simulink model "DroneModelv7_FTX"  (R2025a)
settings: Solver=ode4  StartTime=10  StopTime=60  FixedStep=0.001  RelTol=1e-3
undefined symbols (not defined in the file): ACT_MAP, alpha_vec, alpha_vec_control, beta_vec, bref, Cl0, Clda, Cldr, Cm0, Cmda, Cmde, Cmdr, Cn0, Cnda, Cndr, CX0, CXda, CXde, CXdr, CY0, CYda, CYdr, CZ0, CZda, CZde, CZdr, DEMAND0, DEMAND1, DMP_P, EST_BLEND, EST_P, EST_TS, Kalpha, Kbeta, Kp, Kphi, Kq, Kr, mass, RT_LIM_ALPHA, RT_LIM_BETA, RT_LIM_PHI, RT_PA_SCALE, RT_PB_SCALE, RT_PP_SCALE, RT_SURF_LIM, SENS_P, T_STEP, Tc, x_cg, y_cg, z_cg
libraries: aerolibconvert2 x6, aerolibasang x3, slpidlib x3, aerolibobsolete x1, aerolibadyn x1, aerolibatmos2 x1
Description:
  | DroneModelv7_RT - re-tunable controller, generated by
  | tools/build_rt_v7.m from DroneModelv7_EST.
  | 
  | Adds output limits, clamping anti-windup and surface saturation, and
  | exposes the fixed P gains as scale factors so the loop can be re-tuned
  | against a plant that includes the sensor and estimator models.
  | 
  | Outports 1-13 keep the indices they have in DroneModelv7_EST; 14 and 15
  | are the post-saturation surface deflections. 7 and 8 remain the
  | pre-saturation COMMAND, which is the diagnostic worth keeping.
settings Model: SimulationMode=accelerator  Creator=Avery  LastModifiedBy=avery
settings DataIOCC: ExternalInput=getinputstruct(op1)  InitialState=getstatestruct(op1)
settings OptimizationCC: BlockReduction=off  ConditionallyExecuteInputs=off
settings DebuggingCC: UnconnectedInputMsg=error  UnconnectedOutputMsg=warning  UnconnectedLineMsg=warning
settings RTWCC: GPUComputeCapability=3.5

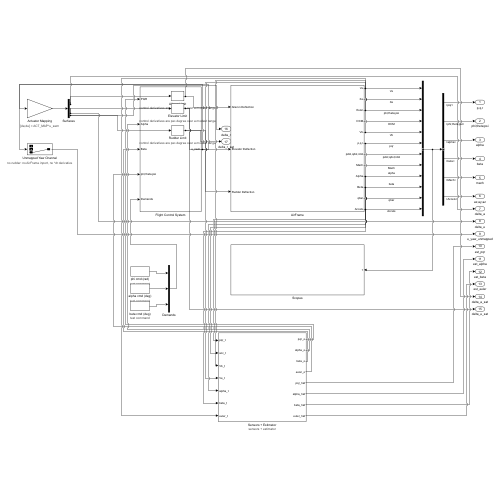
[thumbnail: Simulink's stored preview of the top-level diagram]
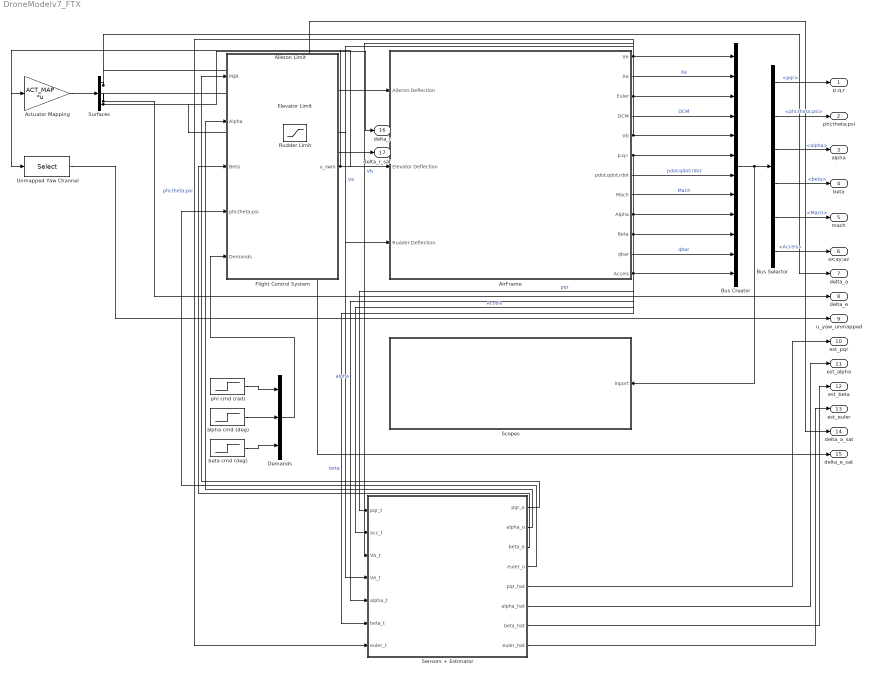
== system DroneModelv7_FTX ==
  Actuator Mapping : Gain  Gain=ACT_MAP  Multiplication=Matrix(K*u)
      settings: AttributesFormatString=[da;de] = ACT_MAP*u_swm
  Aileron Limit : Saturate  UpperLimit=RT_SURF_LIM  LowerLimit=-RT_SURF_LIM
      settings: AttributesFormatString=control derivatives are per-degree over a modest range
  AirFrame : Subsystem
  Bus Creator : BusCreator  Inputs=12
  Bus Selector : BusSelector  OutputSignals=pqr,phi;theta;psi,alpha,beta,Mach,Accels
  Demands : Mux  Inputs=3
  Elevator Limit : Saturate  UpperLimit=RT_SURF_LIM  LowerLimit=-RT_SURF_LIM
      settings: AttributesFormatString=control derivatives are per-degree over a modest range
  Flight Control System : Subsystem
  Rudder Limit : Saturate  UpperLimit=RT_SURF_LIM  LowerLimit=-RT_SURF_LIM
      settings: AttributesFormatString=control derivatives are per-degree over a modest range
  Scopes : Subsystem
  Sensors + Estimator : Subsystem
      settings: AttributesFormatString=sensors + estimator
  Surfaces : Demux  Outputs=3
  Unmapped Yaw Channel : Selector  InputPortWidth=3  IndexOptions=Index vector (dialog)  Indices=[3]  OutputSizes=1
      settings: AttributesFormatString=no rudder: no AirFrame inport, no *dr derivative
  alpha cmd (deg) : Step  Time=T_STEP(2)  Before=DEMAND0(2)  After=DEMAND1(2)  SampleTime=0
      settings: AttributesFormatString=test command
  beta cmd (deg) : Step  Time=T_STEP(3)  Before=DEMAND0(3)  After=DEMAND1(3)  SampleTime=0
      settings: AttributesFormatString=test command
  phi cmd (rad) : Step  Time=T_STEP(1)  Before=DEMAND0(1)  After=DEMAND1(1)  SampleTime=0
      settings: AttributesFormatString=test command
  p,q,r : Outport
  phi;theta;psi : Outport  Port=2
  alpha : Outport  Port=3
  beta : Outport  Port=4
  mach : Outport  Port=5
  ax;ay;az : Outport  Port=6
  delta_a : Outport  Port=7
  delta_e : Outport  Port=8
  u_yaw_unmapped : Outport  Port=9
  est_pqr : Outport  Port=10
  est_alpha : Outport  Port=11
  est_beta : Outport  Port=12
  est_euler : Outport  Port=13
  delta_a_sat : Outport  Port=14
  delta_e_sat : Outport  Port=15
  delta_r : Outport  Port=16
  delta_r_sat : Outport  Port=17
  wires:
  AirFrame/12(Accels) -> Bus Creator/12, Sensors + Estimator/2(acc_t)  "Accels"
  AirFrame/11(qbar) -> Bus Creator/11  "qbar"
  AirFrame/10(Beta) -> Bus Creator/10, Sensors + Estimator/6(beta_t)  "beta"
  AirFrame/9(Alpha) -> Bus Creator/9, Sensors + Estimator/5(alpha_t)  "alpha"
  AirFrame/8(Mach) -> Bus Creator/8  "Mach"
  AirFrame/7(pdot,qdot,rdot) -> Bus Creator/7  "pdot;qdot;rdot"
  AirFrame/6(p,q,r) -> Bus Creator/6, Sensors + Estimator/1(pqr_t)  "pqr"
  AirFrame/5(Vb) -> Bus Creator/5, Sensors + Estimator/3(Vb_t)  "Vb"
  AirFrame/4(DCM) -> Bus Creator/4  "DCM"
  AirFrame/3(Euler) -> Bus Creator/3, Sensors + Estimator/7(euler_t)  "phi;theta;psi"
  AirFrame/2(Xe) -> Bus Creator/2  "Xe"
  AirFrame/1(Ve) -> Bus Creator/1, Sensors + Estimator/4(Ve_t)  "Ve"
  Bus Selector/1 -> p,q,r/1  "<pqr>"
  Bus Selector/2 -> phi;theta;psi/1  "<phi;theta;psi>"
  Bus Selector/3 -> alpha/1  "<alpha>"
  Bus Selector/5 -> mach/1  "<Mach>"
  Bus Selector/6 -> ax;ay;az/1  "<Accels>"
  Bus Selector/4 -> beta/1  "<beta>"
  Bus Creator/1 -> Scopes/1(Inport), Bus Selector/1
  phi cmd (rad)/1 -> Demands/1
  alpha cmd (deg)/1 -> Demands/2
  beta cmd (deg)/1 -> Demands/3
  Demands/1 -> Flight Control System/5(Demands)
  Flight Control System/1(u_swm) -> Actuator Mapping/1, Unmapped Yaw Channel/1
  Actuator Mapping/1 -> Surfaces/1
  Surfaces/1 -> delta_a/1, Aileron Limit/1
  Surfaces/2 -> delta_e/1, Elevator Limit/1
  Unmapped Yaw Channel/1 -> u_yaw_unmapped/1
  Sensors + Estimator/1(pqr_o) -> Flight Control System/1("PQR ")
  Sensors + Estimator/2(alpha_o) -> Flight Control System/2(Alpha)
  Sensors + Estimator/3(beta_o) -> Flight Control System/3(Beta)
  Sensors + Estimator/4(euler_o) -> Flight Control System/4(phi;theta;psi)
  Sensors + Estimator/5(pqr_hat) -> est_pqr/1
  Sensors + Estimator/6(alpha_hat) -> est_alpha/1
  Sensors + Estimator/7(beta_hat) -> est_beta/1
  Sensors + Estimator/8(euler_hat) -> est_euler/1
  Aileron Limit/1 -> AirFrame/1(Aileron Deflection), delta_a_sat/1
  Elevator Limit/1 -> AirFrame/2(Elevator Deflection), delta_e_sat/1
  Surfaces/3 -> Rudder Limit/1, delta_r/1
  Rudder Limit/1 -> AirFrame/3(Rudder Deflection), delta_r_sat/1

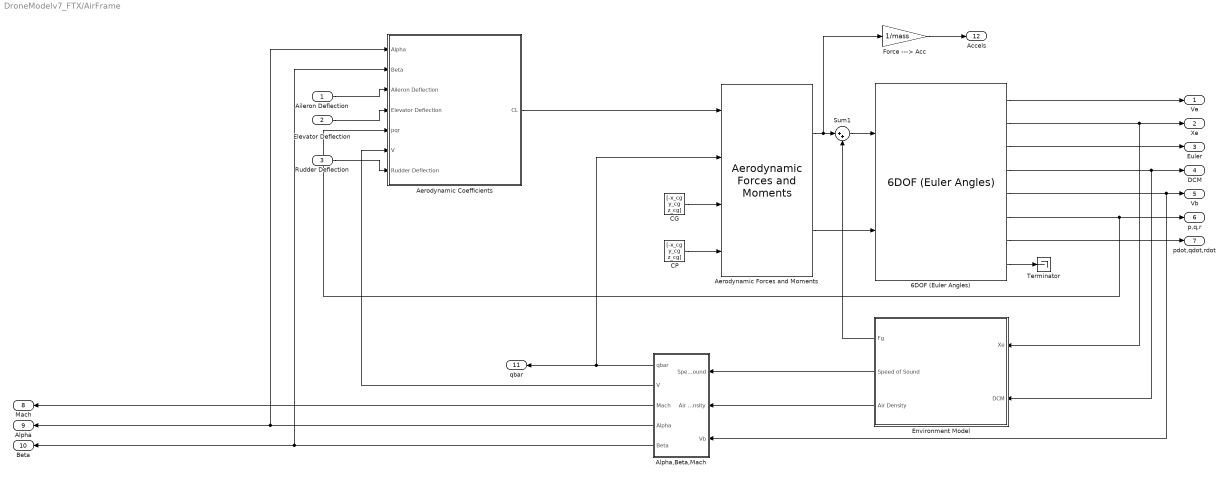
== system DroneModelv7_FTX/AirFrame ==
  Aileron Deflection : Inport  Unit=deg
  Elevator Deflection : Inport  Port=2  Unit=deg
  Rudder Deflection : Inport  Port=3
  6DOF (Euler Angles) : aerolibobsolete/6DOF (Euler Angles)  units=Metric (MKS)  mtype=Fixed  rep=Euler Angles  xme_0=init_pos_inertial  Vm_0=init_velo_body  eul_0=init_euler_orien  pm_0=init_body_rot  mass_0=mass  mass_e=0.5  mass_f=2.0  inertia=Inertia  inertia_e=eye(3)  inertia_f=2*eye(3)  k_quat=1.0  vre_flag=on  abi_flag=off  aMode=0  xme_statename=''  Vm_statename=''  eul_statename=''  quat_statename=''  pm_statename=''  mass_statename=''
  "Aerodynamic Forces and Moments " : aerolibadyn/Aerodynamic Forces and Moments   inputAxes=Body  outputForceAxes=Body  outputMomentAxes=Body  S=Sref  b=bref  cbar=cref
  Aerodynamic Coefficients : Subsystem
  Alpha,Beta,Mach : Subsystem
  CG : Constant  Value=[-x_cg y_cg z_cg]
  CP : Constant  Value=[-x_cg y_cg z_cg]
  Environment Model : Subsystem
  Force ---> Acc : Gain  Gain=1/mass  SaturateOnIntegerOverflow=on  OutDataTypeStr=Inherit: Same as input  ParamDataTypeStr=Inherit: Same as input
  Sum1 : Sum  Inputs=|++  SaturateOnIntegerOverflow=on
  Terminator : Terminator
  Ve : Outport  Unit=m/s
  Xe : Outport  Port=2  Unit=meter
  Euler : Outport  Port=3  Unit=rad
  DCM : Outport  Port=4
  Vb : Outport  Port=5  Unit=m/second
  p,q,r : Outport  Port=6  Unit=rad/second
  pdot,qdot,rdot : Outport  Port=7
  Mach : Outport  Port=8
  Alpha : Outport  Port=9  Unit=rad
  Beta : Outport  Port=10  Unit=rad
  qbar : Outport  Port=11  Unit=Pa
  Accels : Outport  Port=12  Unit=m/s^2
  wires:
  6DOF (Euler Angles)/6 -> Aerodynamic Coefficients/5(pqr), p,q,r/1
  6DOF (Euler Angles)/4 -> DCM/1, Environment Model/2(DCM)
  6DOF (Euler Angles)/2 -> Xe/1, Environment Model/1(Xe)
  6DOF (Euler Angles)/5 -> Alpha,Beta,Mach/3(Vb), Vb/1
  "Aerodynamic Forces and Moments "/1 -> Force ---> Acc/1, Sum1/1
  6DOF (Euler Angles)/3 -> Euler/1
  6DOF (Euler Angles)/1 -> Ve/1
  CP/1 -> "Aerodynamic Forces and Moments "/4
  Alpha,Beta,Mach/1(qbar) -> qbar/1, "Aerodynamic Forces and Moments "/2
  CG/1 -> "Aerodynamic Forces and Moments "/3
  Alpha,Beta,Mach/4(Alpha) -> Aerodynamic Coefficients/1(Alpha), Alpha/1
  6DOF (Euler Angles)/8 -> Terminator/1
  "Aerodynamic Forces and Moments "/2 -> 6DOF (Euler Angles)/2
  6DOF (Euler Angles)/7 -> pdot,qdot,rdot/1
  Alpha,Beta,Mach/2(V) -> Aerodynamic Coefficients/6(V)
  Environment Model/1(Fg) -> Sum1/2
  Sum1/1 -> 6DOF (Euler Angles)/1
  Force ---> Acc/1 -> Accels/1
  Alpha,Beta,Mach/5(Beta) -> Aerodynamic Coefficients/2(Beta), Beta/1
  Alpha,Beta,Mach/3(Mach) -> Mach/1
  Environment Model/2(Speed of Sound) -> Alpha,Beta,Mach/1(Speed of Sound)
  Environment Model/3(Air Density) -> Alpha,Beta,Mach/2(Air Density)
  Aerodynamic Coefficients/1(CL) -> "Aerodynamic Forces and Moments "/1
  Elevator Deflection/1 -> Aerodynamic Coefficients/4(Elevator Deflection)
  Aileron Deflection/1 -> Aerodynamic Coefficients/3(Aileron Deflection)
  Rudder Deflection/1 -> Aerodynamic Coefficients/7(Rudder Deflection)

== system DroneModelv7_FTX/Flight Control System ==
  "PQR " : Inport
  Alpha : Inport  Port=2
  Beta : Inport  Port=3
  phi;theta;psi : Inport  Port=4
  Demands : Inport  Port=5
      settings: AttributesFormatString=test command vector
  Angle Conversion : aerolibconvert2/Angle Conversion  IU=rad  OU=deg
  Angle Conversion1 : aerolibconvert2/Angle Conversion  IU=rad  OU=deg
  Controller : Subsystem
  Selector : Selector  InputPortWidth=3  IndexOptions=Index vector (dialog)  Indices=[1]  OutputSizes=1
  u_swm : Outport
  wires:
  "PQR "/1 -> Controller/5(Rates)
  Alpha/1 -> Angle Conversion/1
  Beta/1 -> Angle Conversion1/1
  Angle Conversion1/1 -> Controller/3(Beta)
  Angle Conversion/1 -> Controller/2(Alpha)
  phi;theta;psi/1 -> Selector/1
  Selector/1 -> Controller/1(Phi)  "phi"
  Demands/1 -> Controller/4(Demands)
  Controller/1(u_swm) -> u_swm/1

== system DroneModelv7_FTX/Scopes ==
  Inport : Inport
  Angle Conversion : aerolibconvert2/Angle Conversion  IU=rad  OU=deg
  Angle Conversion1 : aerolibconvert2/Angle Conversion  IU=rad  OU=deg
  Bus Selector : BusSelector  OutputSignals=alpha,beta,Mach,pqr,phi;theta;psi,Xe,Vb
  Scope : Scope  NumInputPorts=3
      settings: ActiveDisplayYMinimum=2.14483  ActiveDisplayYMaximum=2.82837
  Scope1 : Scope  NumInputPorts=4
      settings: ActiveDisplayYMinimum=-0.1468  ActiveDisplayYMaximum=0.04977
  wires:
  Bus Selector/1 -> Angle Conversion/1  "<alpha>"
  Bus Selector/2 -> Angle Conversion1/1  "<beta>"
  Bus Selector/3 -> Scope/3  "<Mach>"
  Bus Selector/4 -> Scope1/1  "<pqr>"
  Bus Selector/5 -> Scope1/2  "<phi;theta;psi>"
  Bus Selector/6 -> Scope1/3  "<Xe>"
  Inport/1 -> Bus Selector/1
  Angle Conversion1/1 -> Scope/2  "beta"
  Angle Conversion/1 -> Scope/1  "alpha"
  Bus Selector/7 -> Scope1/4  "<Vb>"

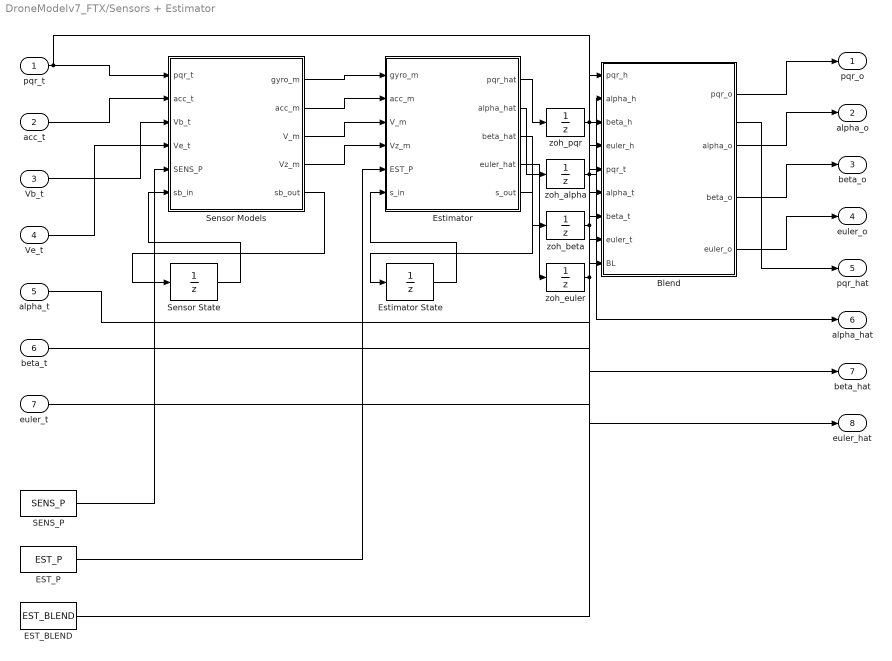
== system DroneModelv7_FTX/Sensors + Estimator ==
  pqr_t : Inport
  acc_t : Inport  Port=2
  Vb_t : Inport  Port=3
  Ve_t : Inport  Port=4
  alpha_t : Inport  Port=5
  beta_t : Inport  Port=6
  euler_t : Inport  Port=7
  Blend : MATLAB Function  TreatAsAtomicUnit=on
  EST_BLEND : Constant  Value=EST_BLEND
  EST_P : Constant  Value=EST_P
  Estimator : MATLAB Function  TreatAsAtomicUnit=on
  Estimator State : UnitDelay  InitialCondition=zeros(10,1)  SampleTime=EST_TS  HasFrameUpgradeWarning=on
  SENS_P : Constant  Value=SENS_P
  Sensor Models : MATLAB Function  TreatAsAtomicUnit=on
  Sensor State : UnitDelay  InitialCondition=zeros(4,1)  SampleTime=EST_TS  HasFrameUpgradeWarning=on
  zoh_alpha : UnitDelay  SampleTime=EST_TS  HasFrameUpgradeWarning=on
      settings: AttributesFormatString=sensor + compute latency, 1 sample
  zoh_beta : UnitDelay  SampleTime=EST_TS  HasFrameUpgradeWarning=on
      settings: AttributesFormatString=sensor + compute latency, 1 sample
  zoh_euler : UnitDelay  SampleTime=EST_TS  HasFrameUpgradeWarning=on
      settings: AttributesFormatString=sensor + compute latency, 1 sample
  zoh_pqr : UnitDelay  SampleTime=EST_TS  HasFrameUpgradeWarning=on
      settings: AttributesFormatString=sensor + compute latency, 1 sample
  pqr_o : Outport
  alpha_o : Outport  Port=2
  beta_o : Outport  Port=3
  euler_o : Outport  Port=4
  pqr_hat : Outport  Port=5
  alpha_hat : Outport  Port=6
  beta_hat : Outport  Port=7
  euler_hat : Outport  Port=8
  wires:
  pqr_t/1 -> Sensor Models/1(pqr_t), Blend/5(pqr_t)
  acc_t/1 -> Sensor Models/2(acc_t)
  Vb_t/1 -> Sensor Models/3(Vb_t)
  Ve_t/1 -> Sensor Models/4(Ve_t)
  SENS_P/1 -> Sensor Models/5(SENS_P)
  Sensor State/1 -> Sensor Models/6(sb_in)
  Sensor Models/5(sb_out) -> Sensor State/1
  Sensor Models/1(gyro_m) -> Estimator/1(gyro_m)
  Sensor Models/2(acc_m) -> Estimator/2(acc_m)
  Sensor Models/3(V_m) -> Estimator/3(V_m)
  Sensor Models/4(Vz_m) -> Estimator/4(Vz_m)
  EST_P/1 -> Estimator/5(EST_P)
  Estimator State/1 -> Estimator/6(s_in)
  Estimator/5(s_out) -> Estimator State/1
  Estimator/1(pqr_hat) -> zoh_pqr/1
  Estimator/2(alpha_hat) -> zoh_alpha/1
  Estimator/3(beta_hat) -> zoh_beta/1
  Estimator/4(euler_hat) -> zoh_euler/1
  zoh_pqr/1 -> Blend/1(pqr_h), pqr_hat/1
  zoh_alpha/1 -> Blend/2(alpha_h), alpha_hat/1
  zoh_beta/1 -> Blend/3(beta_h), beta_hat/1
  zoh_euler/1 -> Blend/4(euler_h), euler_hat/1
  alpha_t/1 -> Blend/6(alpha_t)
  beta_t/1 -> Blend/7(beta_t)
  euler_t/1 -> Blend/8(euler_t)
  EST_BLEND/1 -> Blend/9(BL)
  Blend/1(pqr_o) -> pqr_o/1
  Blend/2(alpha_o) -> alpha_o/1
  Blend/3(beta_o) -> beta_o/1
  Blend/4(euler_o) -> euler_o/1

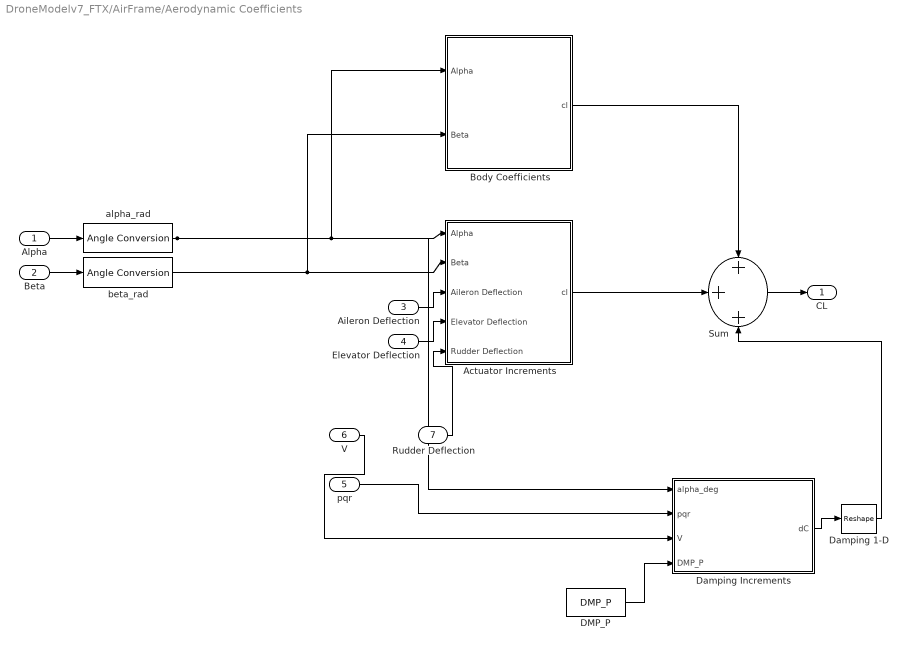
== system DroneModelv7_FTX/AirFrame/Aerodynamic Coefficients ==
  Alpha : Inport
  Beta : Inport  Port=2
  Aileron Deflection : Inport  Port=3
  Elevator Deflection : Inport  Port=4
  pqr : Inport  Port=5
  V : Inport  Port=6
  Rudder Deflection : Inport  Port=7
  Actuator Increments : Subsystem
  Body Coefficients : Subsystem
  DMP_P : Constant  Value=DMP_P
  Damping 1-D : Reshape
  Damping Increments : MATLAB Function  TreatAsAtomicUnit=on
  Sum : Sum  Inputs=+++  InputSameDT=on  SaturateOnIntegerOverflow=on  OutDataTypeStr=Inherit: Same as first input
  alpha_rad : aerolibconvert2/Angle Conversion  IU=rad  OU=deg
  beta_rad : aerolibconvert2/Angle Conversion  IU=rad  OU=deg
  CL : Outport
  wires:
  Elevator Deflection/1 -> Actuator Increments/4(Elevator Deflection)
  Beta/1 -> beta_rad/1
  Alpha/1 -> alpha_rad/1
  Body Coefficients/1(cl) -> Sum/1
  Aileron Deflection/1 -> Actuator Increments/3(Aileron Deflection)
  Actuator Increments/1(cl) -> Sum/2
  Sum/1 -> CL/1
  alpha_rad/1 -> Body Coefficients/1(Alpha), Actuator Increments/1(Alpha), Damping Increments/1(alpha_deg)
  beta_rad/1 -> Body Coefficients/2(Beta), Actuator Increments/2(Beta)
  pqr/1 -> Damping Increments/2(pqr)
  V/1 -> Damping Increments/3(V)
  DMP_P/1 -> Damping Increments/4(DMP_P)
  Damping Increments/1(dC) -> Damping 1-D/1
  Damping 1-D/1 -> Sum/3
  Rudder Deflection/1 -> Actuator Increments/5(Rudder Deflection)

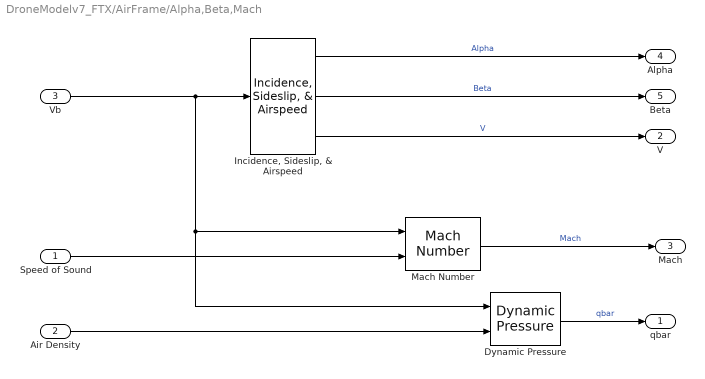
== system DroneModelv7_FTX/AirFrame/Alpha,Beta,Mach ==
  Speed of Sound : Inport
  Air Density : Inport  Port=2
  Vb : Inport  Port=3  PortDimensions=3
  Dynamic Pressure : aerolibasang/Dynamic Pressure
  "Incidence, Sideslip, & Airspeed" : aerolibasang/Incidence, Sideslip, & Airspeed
  Mach Number : aerolibasang/Mach Number
  qbar : Outport  Unit=Pa  InitialOutput=0  VectorParamsAs1DForOutWhenUnconnected=off
  V : Outport  Port=2  Unit=m/s  VectorParamsAs1DForOutWhenUnconnected=off
  Mach : Outport  Port=3  VectorParamsAs1DForOutWhenUnconnected=off
  Alpha : Outport  Port=4  Unit=rad  VectorParamsAs1DForOutWhenUnconnected=off
  Beta : Outport  Port=5  Unit=rad  VectorParamsAs1DForOutWhenUnconnected=off
  wires:
  Air Density/1 -> Dynamic Pressure/2
  "Incidence, Sideslip, & Airspeed"/2 -> Beta/1  "Beta"
  "Incidence, Sideslip, & Airspeed"/1 -> Alpha/1  "Alpha"
  Vb/1 -> Dynamic Pressure/1, Mach Number/1, "Incidence, Sideslip, & Airspeed"/1
  Mach Number/1 -> Mach/1  "Mach"
  Dynamic Pressure/1 -> qbar/1  "qbar"
  Speed of Sound/1 -> Mach Number/2
  "Incidence, Sideslip, & Airspeed"/3 -> V/1  "V"

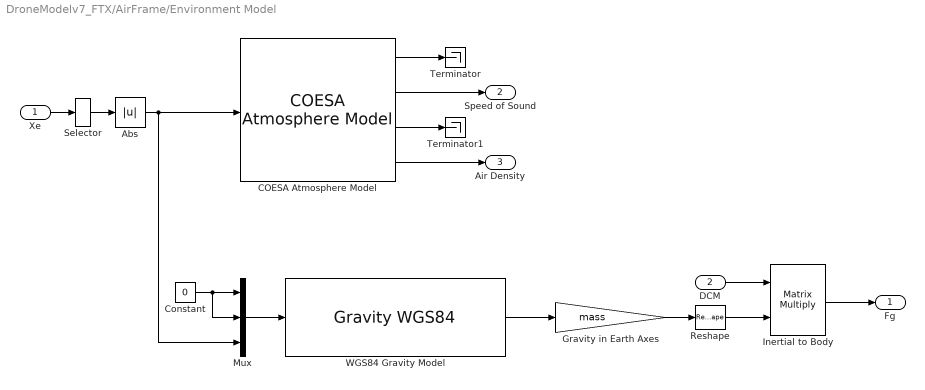
== system DroneModelv7_FTX/AirFrame/Environment Model ==
  Xe : Inport  Unit=meter  PortDimensions=3
  DCM : Inport  Port=2
  Abs : Abs  SaturateOnIntegerOverflow=off
  COESA Atmosphere Model : aerolibatmos2/COESA Atmosphere Model  units=Metric (MKS)  spec=1976 COESA-extended U.S. Standard Atmosphere  model=Profile  profile_var=High temperature  profile_percent=1%  profile_alt=5 km (16404 ft)  envelope_var=High temperature  envelope_percent=1%  action=Warning
  Constant : Constant  Value=0
  Gravity in Earth Axes : Gain  Gain=mass  SaturateOnIntegerOverflow=on  ParamDataTypeStr=Inherit: Same as input
  Inertial to Body : Product  Multiplication=Matrix(*)  InputSameDT=on  SaturateOnIntegerOverflow=on  OutDataTypeStr=Inherit: Same as first input
  Mux : Mux  Inputs=3
  Reshape : Reshape
  Selector : Selector  InputPortWidth=3  IndexOptions=Index vector (dialog)  Indices=[3]  OutputSizes=1
  Terminator : Terminator
  Terminator1 : Terminator
  "WGS84 Gravity Model  " : GravityWGS84  action=None
  Fg : Outport
  Speed of Sound : Outport  Port=2
  Air Density : Outport  Port=3
  wires:
  COESA Atmosphere Model/1 -> Terminator/1
  COESA Atmosphere Model/3 -> Terminator1/1
  COESA Atmosphere Model/2 -> Speed of Sound/1
  COESA Atmosphere Model/4 -> Air Density/1
  Reshape/1 -> Inertial to Body/2
  Gravity in Earth Axes/1 -> Reshape/1
  DCM/1 -> Inertial to Body/1
  Inertial to Body/1 -> Fg/1
  Abs/1 -> Mux/3, COESA Atmosphere Model/1
  Constant/1 -> Mux/1, Mux/2
  Mux/1 -> "WGS84 Gravity Model  "/1
  "WGS84 Gravity Model  "/1 -> Gravity in Earth Axes/1
  Xe/1 -> Selector/1
  Selector/1 -> Abs/1

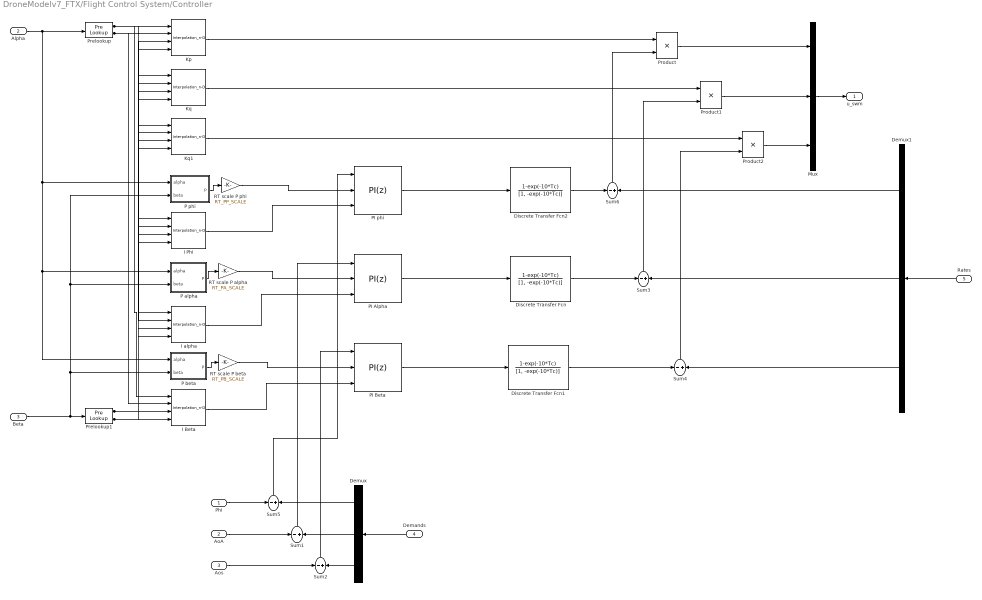
== system DroneModelv7_FTX/Flight Control System/Controller ==
  Phi : Inport
  Alpha : Inport  Port=2
  Beta : Inport  Port=3
  Demands : Inport  Port=4
  Rates : Inport  Port=5
  AoA : InportShadow  Port=2
  Aos : InportShadow  Port=3
  Demux : Demux  Outputs=3
  Demux1 : Demux  Outputs=3
  Discrete Transfer Fcn : DiscreteTransferFcn  Numerator=1-exp(-10*Tc)  Denominator=[1, -exp(-10*Tc)]  SampleTime=Tc  SaturateOnIntegerOverflow=on
      settings: AttributesFormatString=ZOH of 10/(s+10) as an expression in Tc
  Discrete Transfer Fcn1 : DiscreteTransferFcn  Numerator=1-exp(-10*Tc)  Denominator=[1, -exp(-10*Tc)]  SampleTime=Tc  SaturateOnIntegerOverflow=on
      settings: AttributesFormatString=ZOH of 10/(s+10) as an expression in Tc
  Discrete Transfer Fcn2 : DiscreteTransferFcn  Numerator=1-exp(-10*Tc)  Denominator=[1, -exp(-10*Tc)]  SampleTime=Tc  SaturateOnIntegerOverflow=on
      settings: AttributesFormatString=ZOH of 10/(s+10) as an expression in Tc
  I Beta : Interpolation_n-D  Table=Kbeta  RemoveProtectionIndex=on
  I Phi : Interpolation_n-D  Table=Kphi  RemoveProtectionIndex=on
  I alpha : Interpolation_n-D  Table=Kalpha  RemoveProtectionIndex=on
  Kp : Interpolation_n-D  Table=Kp  RemoveProtectionIndex=on
  Kq : Interpolation_n-D  Table=Kq  RemoveProtectionIndex=on
  Kq1 : Interpolation_n-D  Table=Kr  RemoveProtectionIndex=on
  Mux : Mux  Inputs=3
  P alpha : MATLAB Function  TreatAsAtomicUnit=on
  P beta : MATLAB Function  TreatAsAtomicUnit=on
  P phi : MATLAB Function  TreatAsAtomicUnit=on
  PI Alpha : slpidlib/PID Controller  Controller=PI  Form=Parallel  TimeDomain=Discrete-time  UseExternalTs=off  SampleTime=Tc  IntegratorMethod=Forward Euler  FilterMethod=Forward Euler  ControllerParametersSource=external  P=1  I=1  UseKiTs=off  D=0  N=100  UseFilter=on  TunerSelectOption=Transfer Function Based (PID Tuner App)  InitialConditionSource=internal  InitialConditionForIntegrator=0  InitialConditionForFilter=0  DifferentiatorICPrevScaledInput=0  ExternalReset=none  TrackingMode=off  Kt=1  LimitOutput=on  SatLimitsSource=internal  UpperSaturationLimit=RT_LIM_ALPHA  LowerSaturationLimit=-RT_LIM_ALPHA  LinearizeAsGain=on  AntiWindupMode=clamping  Kb=1  LimitIntegrator=off  UpperIntegratorSaturationLimit=inf  LowerIntegratorSaturationLimit=-inf  POutMin=[]  POutMax=[]  IOutMin=[]  IOutMax=[]  DOutMin=[]  DOutMax=[]  NOutMin=[]  NOutMax=[]  SumOutMin=[]  SumOutMax=[]  SaturationOutMin=[]  SaturationOutMax=[]  PParamMin=[]  PParamMax=[]  IParamMin=[]  IParamMax=[]  DParamMin=[]  DParamMax=[]  NParamMin=[]  NParamMax=[]  KbParamMin=[]  KbParamMax=[]  KtParamMin=[]  KtParamMax=[]  KbOutMin=[]  KbOutMax=[]  KtOutMin=[]  KtOutMax=[]  IntegratorOutMin=[]  IntegratorOutMax=[]  FilterOutMin=[]  FilterOutMax=[]  SumI1OutMin=[]  SumI1OutMax=[]  SumI2OutMin=[]  SumI2OutMax=[]  SumI3OutMin=[]  SumI3OutMax=[]  SumI4OutMin=[]  SumI4OutMax=[]  SumDOutMin=[]  SumDOutMax=[]  DifferentiatorOutMin=[]  DifferentiatorOutMax=[]  FilterDiffOutCoefMin=[]  FilterDiffOutCoefMax=[]  ReciprocalOutMin=[]  ReciprocalOutMax=[]  SumDenOutMin=[]  SumDenOutMax=[]  SumNumOutMin=[]  SumNumOutMax=[]  DivideOutMin=[]  DivideOutMax=[]  UdiffTsProdOutMin=[]  UdiffTsProdOutMax=[]  NTsProdOutMin=[]  NTsProdOutMax=[]  UintegralTsProdOutMin=[]  UintegralTsProdOutMax=[]  UngainTsProdOutMin=[]  UngainTsProdOutMax=[]  ClampingZeroOutDataTypeStr=Inherit: Inherit via back propagation  ClampingZeroOutMin=[]  ClampingZeroOutMax=[]  FilterDenConstantOutDataTypeStr=Inherit: Inherit via back propagation  FilterDenConstantOutMin=[]  FilterDenConstantOutMax=[]  PCopyOutDataTypeStr=Inherit: Inherit via back propagation  PCopyOutMin=[]  PCopyOutMax=[]  NCopyOutDataTypeStr=Inherit: Inherit via back propagation  NCopyOutMin=[]  NCopyOutMax=[]  IntegratorContinuousStateAttributes=''  IntegratorStateMustResolveToSignalObject=off  IntegratorRTWStateStorageClass=Auto  FilterContinuousStateAttributes=''  FilterStateMustResolveToSignalObject=off  FilterRTWStateStorageClass=Auto  ParallelPVariant=ExternalParameters  IdealPVariant=Disabled  IVariant=ExternalParameters  DVariant=Disabled  IntegratorVariant=Discrete  SatVariant=Enabled  AWVariant=DiscClampingParallel  PCopyVariant=Disabled  TRVariant=Disabled  FdbkBlocksVariant=Forward  IdealPFdbkVariant=Disabled  SatFdbkVariant=Disabled  DerivativeFilterVariant=Disabled  NVariant=Disabled  NCopyVariant=Disabled_SignalSpec  FilterICVariant=Disabled  IntegratorICVariant=InternalICs  ExternalResetVariant=Disabled  TRSumVariant=Passthrough  SumFdbkVariant=Disabled  SumVariant=Sum_PI  TsampFilterVariant=InternalTs  TsampNgainVariant=Passthrough  TsampIntegralVariant=Disabled_SignalSpec  ExternalSaturationOutDataTypeStr=Inherit: Same as second input
      settings: AttributesFormatString=output limited to +-RT_LIM_ALPHA, clamping anti-windup
  PI Beta : slpidlib/PID Controller  Controller=PI  Form=Parallel  TimeDomain=Discrete-time  UseExternalTs=off  SampleTime=Tc  IntegratorMethod=Forward Euler  FilterMethod=Forward Euler  ControllerParametersSource=external  P=1  I=1  UseKiTs=off  D=0  N=100  UseFilter=on  TunerSelectOption=Transfer Function Based (PID Tuner App)  InitialConditionSource=internal  InitialConditionForIntegrator=0  InitialConditionForFilter=0  DifferentiatorICPrevScaledInput=0  ExternalReset=none  TrackingMode=off  Kt=1  LimitOutput=on  SatLimitsSource=internal  UpperSaturationLimit=RT_LIM_BETA  LowerSaturationLimit=-RT_LIM_BETA  LinearizeAsGain=on  AntiWindupMode=clamping  Kb=1  LimitIntegrator=off  UpperIntegratorSaturationLimit=inf  LowerIntegratorSaturationLimit=-inf  POutMin=[]  POutMax=[]  IOutMin=[]  IOutMax=[]  DOutMin=[]  DOutMax=[]  NOutMin=[]  NOutMax=[]  SumOutMin=[]  SumOutMax=[]  SaturationOutMin=[]  SaturationOutMax=[]  PParamMin=[]  PParamMax=[]  IParamMin=[]  IParamMax=[]  DParamMin=[]  DParamMax=[]  NParamMin=[]  NParamMax=[]  KbParamMin=[]  KbParamMax=[]  KtParamMin=[]  KtParamMax=[]  KbOutMin=[]  KbOutMax=[]  KtOutMin=[]  KtOutMax=[]  IntegratorOutMin=[]  IntegratorOutMax=[]  FilterOutMin=[]  FilterOutMax=[]  SumI1OutMin=[]  SumI1OutMax=[]  SumI2OutMin=[]  SumI2OutMax=[]  SumI3OutMin=[]  SumI3OutMax=[]  SumI4OutMin=[]  SumI4OutMax=[]  SumDOutMin=[]  SumDOutMax=[]  DifferentiatorOutMin=[]  DifferentiatorOutMax=[]  FilterDiffOutCoefMin=[]  FilterDiffOutCoefMax=[]  ReciprocalOutMin=[]  ReciprocalOutMax=[]  SumDenOutMin=[]  SumDenOutMax=[]  SumNumOutMin=[]  SumNumOutMax=[]  DivideOutMin=[]  DivideOutMax=[]  UdiffTsProdOutMin=[]  UdiffTsProdOutMax=[]  NTsProdOutMin=[]  NTsProdOutMax=[]  UintegralTsProdOutMin=[]  UintegralTsProdOutMax=[]  UngainTsProdOutMin=[]  UngainTsProdOutMax=[]  ClampingZeroOutDataTypeStr=Inherit: Inherit via back propagation  ClampingZeroOutMin=[]  ClampingZeroOutMax=[]  FilterDenConstantOutDataTypeStr=Inherit: Inherit via back propagation  FilterDenConstantOutMin=[]  FilterDenConstantOutMax=[]  PCopyOutDataTypeStr=Inherit: Inherit via back propagation  PCopyOutMin=[]  PCopyOutMax=[]  NCopyOutDataTypeStr=Inherit: Inherit via back propagation  NCopyOutMin=[]  NCopyOutMax=[]  IntegratorContinuousStateAttributes=''  IntegratorStateMustResolveToSignalObject=off  IntegratorRTWStateStorageClass=Auto  FilterContinuousStateAttributes=''  FilterStateMustResolveToSignalObject=off  FilterRTWStateStorageClass=Auto  ParallelPVariant=ExternalParameters  IdealPVariant=Disabled  IVariant=ExternalParameters  DVariant=Disabled  IntegratorVariant=Discrete  SatVariant=Enabled  AWVariant=DiscClampingParallel  PCopyVariant=Disabled  TRVariant=Disabled  FdbkBlocksVariant=Forward  IdealPFdbkVariant=Disabled  SatFdbkVariant=Disabled  DerivativeFilterVariant=Disabled  NVariant=Disabled  NCopyVariant=Disabled_SignalSpec  FilterICVariant=Disabled  IntegratorICVariant=InternalICs  ExternalResetVariant=Disabled  TRSumVariant=Passthrough  SumFdbkVariant=Disabled  SumVariant=Sum_PI  TsampFilterVariant=InternalTs  TsampNgainVariant=Passthrough  TsampIntegralVariant=Disabled_SignalSpec  ExternalSaturationOutDataTypeStr=Inherit: Same as second input
      settings: AttributesFormatString=output limited to +-RT_LIM_BETA, clamping anti-windup
  PI phi : slpidlib/PID Controller  Controller=PI  Form=Parallel  TimeDomain=Discrete-time  UseExternalTs=off  SampleTime=Tc  IntegratorMethod=Forward Euler  FilterMethod=Forward Euler  ControllerParametersSource=external  P=1  I=1  UseKiTs=off  D=0  N=100  UseFilter=on  TunerSelectOption=Transfer Function Based (PID Tuner App)  InitialConditionSource=internal  InitialConditionForIntegrator=0  InitialConditionForFilter=0  DifferentiatorICPrevScaledInput=0  ExternalReset=none  TrackingMode=off  Kt=1  LimitOutput=on  SatLimitsSource=internal  UpperSaturationLimit=RT_LIM_PHI  LowerSaturationLimit=-RT_LIM_PHI  LinearizeAsGain=on  AntiWindupMode=clamping  Kb=1  LimitIntegrator=off  UpperIntegratorSaturationLimit=inf  LowerIntegratorSaturationLimit=-inf  POutMin=[]  POutMax=[]  IOutMin=[]  IOutMax=[]  DOutMin=[]  DOutMax=[]  NOutMin=[]  NOutMax=[]  SumOutMin=[]  SumOutMax=[]  SaturationOutMin=[]  SaturationOutMax=[]  PParamMin=[]  PParamMax=[]  IParamMin=[]  IParamMax=[]  DParamMin=[]  DParamMax=[]  NParamMin=[]  NParamMax=[]  KbParamMin=[]  KbParamMax=[]  KtParamMin=[]  KtParamMax=[]  KbOutMin=[]  KbOutMax=[]  KtOutMin=[]  KtOutMax=[]  IntegratorOutMin=[]  IntegratorOutMax=[]  FilterOutMin=[]  FilterOutMax=[]  SumI1OutMin=[]  SumI1OutMax=[]  SumI2OutMin=[]  SumI2OutMax=[]  SumI3OutMin=[]  SumI3OutMax=[]  SumI4OutMin=[]  SumI4OutMax=[]  SumDOutMin=[]  SumDOutMax=[]  DifferentiatorOutMin=[]  DifferentiatorOutMax=[]  FilterDiffOutCoefMin=[]  FilterDiffOutCoefMax=[]  ReciprocalOutMin=[]  ReciprocalOutMax=[]  SumDenOutMin=[]  SumDenOutMax=[]  SumNumOutMin=[]  SumNumOutMax=[]  DivideOutMin=[]  DivideOutMax=[]  UdiffTsProdOutMin=[]  UdiffTsProdOutMax=[]  NTsProdOutMin=[]  NTsProdOutMax=[]  UintegralTsProdOutMin=[]  UintegralTsProdOutMax=[]  UngainTsProdOutMin=[]  UngainTsProdOutMax=[]  ClampingZeroOutDataTypeStr=Inherit: Inherit via back propagation  ClampingZeroOutMin=[]  ClampingZeroOutMax=[]  FilterDenConstantOutDataTypeStr=Inherit: Inherit via back propagation  FilterDenConstantOutMin=[]  FilterDenConstantOutMax=[]  PCopyOutDataTypeStr=Inherit: Inherit via back propagation  PCopyOutMin=[]  PCopyOutMax=[]  NCopyOutDataTypeStr=Inherit: Inherit via back propagation  NCopyOutMin=[]  NCopyOutMax=[]  IntegratorContinuousStateAttributes=''  IntegratorStateMustResolveToSignalObject=off  IntegratorRTWStateStorageClass=Auto  FilterContinuousStateAttributes=''  FilterStateMustResolveToSignalObject=off  FilterRTWStateStorageClass=Auto  ParallelPVariant=ExternalParameters  IdealPVariant=Disabled  IVariant=ExternalParameters  DVariant=Disabled  IntegratorVariant=Discrete  SatVariant=Enabled  AWVariant=DiscClampingParallel  PCopyVariant=Disabled  TRVariant=Disabled  FdbkBlocksVariant=Forward  IdealPFdbkVariant=Disabled  SatFdbkVariant=Disabled  DerivativeFilterVariant=Disabled  NVariant=Disabled  NCopyVariant=Disabled_SignalSpec  FilterICVariant=Disabled  IntegratorICVariant=InternalICs  ExternalResetVariant=Disabled  TRSumVariant=Passthrough  SumFdbkVariant=Disabled  SumVariant=Sum_PI  TsampFilterVariant=InternalTs  TsampNgainVariant=Passthrough  TsampIntegralVariant=Disabled_SignalSpec  ExternalSaturationOutDataTypeStr=Inherit: Same as second input
      settings: AttributesFormatString=output limited to +-RT_LIM_PHI, clamping anti-windup
  Prelookup : PreLookup  BreakpointsData=a_vec  BeginIndexSearchUsingPreviousIndexResult=on  ExtrapMethod=Linear
  Prelookup1 : PreLookup  BreakpointsData=b_vec  BeginIndexSearchUsingPreviousIndexResult=on  ExtrapMethod=Linear
  Product : Product
  Product1 : Product
  Product2 : Product
  RT scale P alpha : Gain  Gain=RT_PA_SCALE
      settings: AttributesFormatString=retune handle on the fixed P alpha gain
  RT scale P beta : Gain  Gain=RT_PB_SCALE
      settings: AttributesFormatString=retune handle on the fixed P beta gain
  RT scale P phi : Gain  Gain=RT_PP_SCALE
      settings: AttributesFormatString=retune handle on the fixed P phi gain
  Sum{1..6} (6 alike) : Sum  Inputs=-|+
  u_swm : Outport
  wires:
  Alpha/1 -> P phi/1(alpha), P beta/1(alpha), P alpha/1(alpha), Prelookup/1
  Prelookup/1 -> I Phi/1, I alpha/1, Kp/1, I Beta/1, Kq/1, Kq1/1
  Prelookup/2 -> I Phi/2, I alpha/2, Kp/2, I Beta/2, Kq/2, Kq1/2
  Beta/1 -> P phi/2(beta), P alpha/2(beta), P beta/2(beta), Prelookup1/1
  Prelookup1/1 -> I Beta/3, I Phi/3, I alpha/3, Kp/3, Kq/3, Kq1/3
  Prelookup1/2 -> I Phi/4, I alpha/4, Kp/4, I Beta/4, Kq/4, Kq1/4
  Aos/1 -> Sum2/1
  AoA/1 -> Sum1/1
  Demands/1 -> Demux/1
  Sum1/1 -> PI Alpha/1
  Sum2/1 -> PI Beta/1
  I Beta/1 -> PI Beta/3
  I alpha/1 -> PI Alpha/3
  PI Alpha/1 -> Discrete Transfer Fcn/1
  Discrete Transfer Fcn/1 -> Sum3/1
  Discrete Transfer Fcn1/1 -> Sum4/1
  I Phi/1 -> PI phi/3
  Demux/3 -> Sum2/2
  Demux/2 -> Sum1/2
  Phi/1 -> Sum5/1
  Demux/1 -> Sum5/2
  Sum5/1 -> PI phi/1
  PI phi/1 -> Discrete Transfer Fcn2/1
  Discrete Transfer Fcn2/1 -> Sum6/1
  Kp/1 -> Product/1
  Kq/1 -> Product1/1
  Kq1/1 -> Product2/1
  Sum6/1 -> Product/2
  Sum3/1 -> Product1/2
  Sum4/1 -> Product2/2
  PI Beta/1 -> Discrete Transfer Fcn1/1
  Product/1 -> Mux/1
  Product1/1 -> Mux/2
  Product2/1 -> Mux/3
  Mux/1 -> u_swm/1
  Demux1/1 -> Sum6/2
  Demux1/2 -> Sum3/2
  Demux1/3 -> Sum4/2
  Rates/1 -> Demux1/1
  P alpha/1(P) -> RT scale P alpha/1
  RT scale P alpha/1 -> PI Alpha/2
  P beta/1(P) -> RT scale P beta/1
  RT scale P beta/1 -> PI Beta/2
  P phi/1(P) -> RT scale P phi/1
  RT scale P phi/1 -> PI phi/2

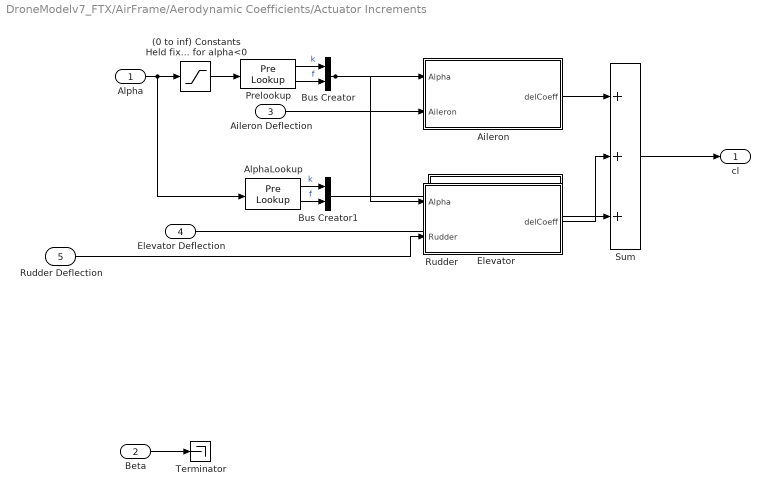
== system DroneModelv7_FTX/AirFrame/Aerodynamic Coefficients/Actuator Increments ==
  Alpha : Inport
  Beta : Inport  Port=2
  Aileron Deflection : Inport  Port=3
  Elevator Deflection : Inport  Port=4
  Rudder Deflection : Inport  Port=5
  (0 to inf) Constants Held fixed for alpha<0 : Saturate  UpperLimit=alpha_vec_control(end)  LowerLimit=alpha_vec_control(1)
  Aileron : Subsystem  AncestorBlock=|
      | aeroblk_lib_HL20/HL20
      | Airframe/Aerodynamic
      | Coefficients/Actuator
      | Increments/Aileron
  AlphaLookup : PreLookup  BreakpointsData=alpha_vec_control  BeginIndexSearchUsingPreviousIndexResult=on  ExtrapMethod=Linear
  Bus Creator : BusCreator  Inputs=2
  Bus Creator1 : BusCreator  Inputs=2
  Elevator : Subsystem  AncestorBlock=|
      | aeroblk_lib_HL20/HL20
      | Airframe/Aerodynamic
      | Coefficients/Actuator
      | Increments/Elevator
  Prelookup : PreLookup  BreakpointsData=alpha_vec_control  BeginIndexSearchUsingPreviousIndexResult=on  ExtrapMethod=Linear
  Rudder : Subsystem  AncestorBlock=|
      | aeroblk_lib_HL20/HL20
      | Airframe/Aerodynamic
      | Coefficients/Actuator
      | Increments/Aileron
  Sum : Sum  Inputs=+++  InputSameDT=on  SaturateOnIntegerOverflow=on
  Terminator : Terminator
  cl : Outport
  wires:
  Beta/1 -> Terminator/1
  Alpha/1 -> AlphaLookup/1, (0 to inf) Constants Held fixed for alpha<0/1
  (0 to inf) Constants Held fixed for alpha<0/1 -> Prelookup/1
  Prelookup/1 -> Bus Creator/1  "k"
  Prelookup/2 -> Bus Creator/2  "f"
  Bus Creator/1 -> Aileron/1(Alpha), Rudder/1(Alpha)
  AlphaLookup/1 -> Bus Creator1/1  "k"
  AlphaLookup/2 -> Bus Creator1/2  "f"
  Bus Creator1/1 -> Elevator/1(Alpha)
  Elevator/1(delCoeff) -> Sum/2
  Aileron/1(delCoeff) -> Sum/1
  Sum/1 -> cl/1
  Elevator Deflection/1 -> Elevator/2(Elevator)
  Aileron Deflection/1 -> Aileron/2(Aileron)
  Rudder Deflection/1 -> Rudder/2(Rudder)
  Rudder/1(delCoeff) -> Sum/3

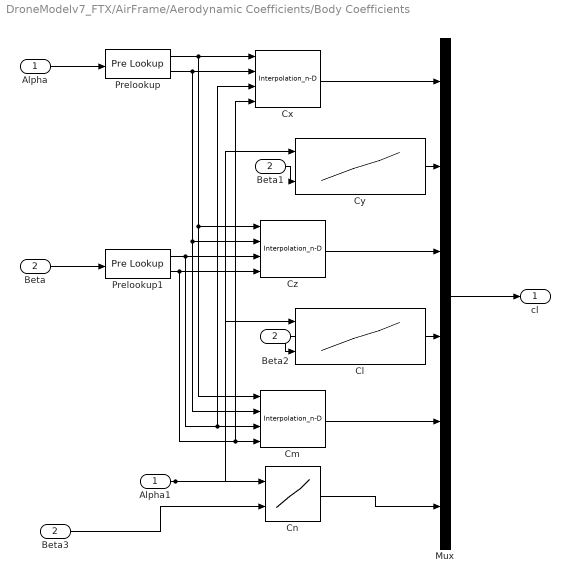
== system DroneModelv7_FTX/AirFrame/Aerodynamic Coefficients/Body Coefficients ==
  Alpha : Inport
  Beta : Inport  Port=2
  " Cn" : Lookup_n-D  BreakpointsForDimension1=alpha_vec  BreakpointsForDimension2=beta_vec  Table=Cn0  InternalRulePriority=Speed  RndMeth=Simplest
      settings: InputPortMap=u0,u1
  Alpha1 : InportShadow
  Beta1 : InportShadow  Port=2
  Beta2 : InportShadow  Port=2
  Beta3 : InportShadow  Port=2
  Cl : Lookup_n-D  BreakpointsForDimension1=alpha_vec  BreakpointsForDimension2=beta_vec  BreakpointsForDimension3=[5, 7]  Table=Cl0  InternalRulePriority=Speed  RndMeth=Simplest
      settings: InputPortMap=u0,u1
  Cm : Interpolation_n-D  Table=Cm0  RemoveProtectionIndex=on  SaturateOnIntegerOverflow=on
  Cx : Interpolation_n-D  Table=CX0  RemoveProtectionIndex=on  SaturateOnIntegerOverflow=on
  Cy : Lookup_n-D  BreakpointsForDimension1=alpha_vec  BreakpointsForDimension2=beta_vec  BreakpointsForDimension3=[5, 7]  Table=CY0  InternalRulePriority=Speed  RndMeth=Simplest
      settings: InputPortMap=u0,u1
  Cz : Interpolation_n-D  Table=CZ0  RemoveProtectionIndex=on  SaturateOnIntegerOverflow=on
  Mux : Mux  Inputs=6
  Prelookup : PreLookup  BreakpointsData=alpha_vec  BeginIndexSearchUsingPreviousIndexResult=on  ExtrapMethod=Linear
  Prelookup1 : PreLookup  BreakpointsData=beta_vec  BeginIndexSearchUsingPreviousIndexResult=on  ExtrapMethod=Linear
  cl : Outport
  wires:
  Alpha/1 -> Prelookup/1
  Prelookup/1 -> Cx/1, Cm/1, Cz/1
  Prelookup/2 -> Cx/2, Cm/2, Cz/2
  Prelookup1/1 -> Cx/3, Cm/3, Cz/3
  Prelookup1/2 -> Cx/4, Cm/4, Cz/4
  Beta/1 -> Prelookup1/1
  Alpha1/1 -> " Cn"/1, Cy/1, Cl/1
  Cz/1 -> Mux/3
  Cx/1 -> Mux/1
  Cm/1 -> Mux/5
  Mux/1 -> cl/1
  Beta3/1 -> " Cn"/2
  " Cn"/1 -> Mux/6
  Beta1/1 -> Cy/2
  Cy/1 -> Mux/2
  Beta2/1 -> Cl/2
  Cl/1 -> Mux/4

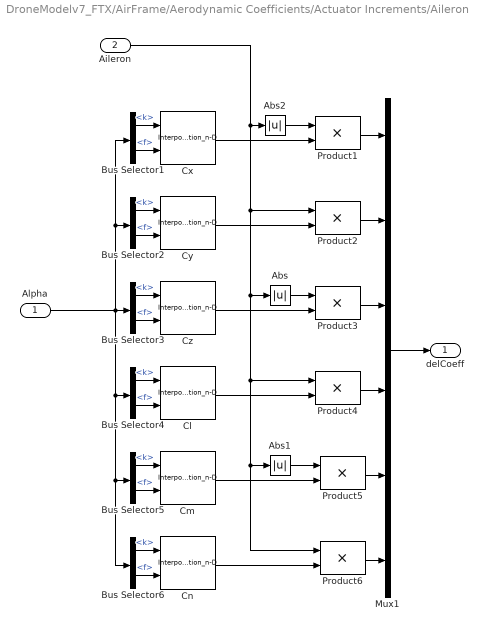
== system DroneModelv7_FTX/AirFrame/Aerodynamic Coefficients/Actuator Increments/Aileron ==
  Alpha : Inport
  Aileron : Inport  Port=2
  Abs : Abs
  Abs1 : Abs
  Abs2 : Abs
  Bus Selector{1..6} (6 alike) : BusSelector  OutputSignals=k,f
  Cl : Interpolation_n-D  NumberOfTableDimensions=1  Table=Clda  RemoveProtectionIndex=on  SaturateOnIntegerOverflow=on
      settings: InputPortMap=u0,u1
  Cm : Interpolation_n-D  NumberOfTableDimensions=1  Table=Cmda  RemoveProtectionIndex=on  SaturateOnIntegerOverflow=on
      settings: InputPortMap=u0,u1
  Cn : Interpolation_n-D  NumberOfTableDimensions=1  Table=Cnda  RemoveProtectionIndex=on  SaturateOnIntegerOverflow=on
      settings: InputPortMap=u0,u1
  Cx : Interpolation_n-D  NumberOfTableDimensions=1  Table=CXda  RemoveProtectionIndex=on  SaturateOnIntegerOverflow=on
      settings: InputPortMap=u0,u1
  Cy : Interpolation_n-D  NumberOfTableDimensions=1  Table=CYda  RemoveProtectionIndex=on  SaturateOnIntegerOverflow=on
      settings: InputPortMap=u0,u1
  Cz : Interpolation_n-D  NumberOfTableDimensions=1  Table=CZda  RemoveProtectionIndex=on  SaturateOnIntegerOverflow=on
      settings: InputPortMap=u0,u1
  Mux1 : Mux  Inputs=6
  Product{1..6} (6 alike) : Product  InputSameDT=on  SaturateOnIntegerOverflow=on  OutDataTypeStr=Inherit: Same as first input
  delCoeff : Outport  VectorParamsAs1DForOutWhenUnconnected=off
  wires:
  Bus Selector6/2 -> Cn/2  "<f>"
  Bus Selector6/1 -> Cn/1  "<k>"
  Bus Selector5/2 -> Cm/2  "<f>"
  Bus Selector5/1 -> Cm/1  "<k>"
  Bus Selector4/2 -> Cl/2  "<f>"
  Bus Selector4/1 -> Cl/1  "<k>"
  Bus Selector3/2 -> Cz/2  "<f>"
  Bus Selector3/1 -> Cz/1  "<k>"
  Bus Selector2/2 -> Cy/2  "<f>"
  Bus Selector2/1 -> Cy/1  "<k>"
  Bus Selector1/2 -> Cx/2  "<f>"
  Bus Selector1/1 -> Cx/1  "<k>"
  Alpha/1 -> Bus Selector3/1, Bus Selector4/1, Bus Selector6/1, Bus Selector5/1, Bus Selector2/1, Bus Selector1/1
  Abs2/1 -> Product1/1
  Abs1/1 -> Product5/1
  Abs/1 -> Product3/1
  Aileron/1 -> Abs2/1, Product2/1, Abs/1, Product4/1, Abs1/1, Product6/1
  Product6/1 -> Mux1/6
  Cn/1 -> Product6/2
  Product5/1 -> Mux1/5
  Cm/1 -> Product5/2
  Product4/1 -> Mux1/4
  Cl/1 -> Product4/2
  Cz/1 -> Product3/2
  Product3/1 -> Mux1/3
  Cy/1 -> Product2/2
  Product2/1 -> Mux1/2
  Cx/1 -> Product1/2
  Product1/1 -> Mux1/1
  Mux1/1 -> delCoeff/1

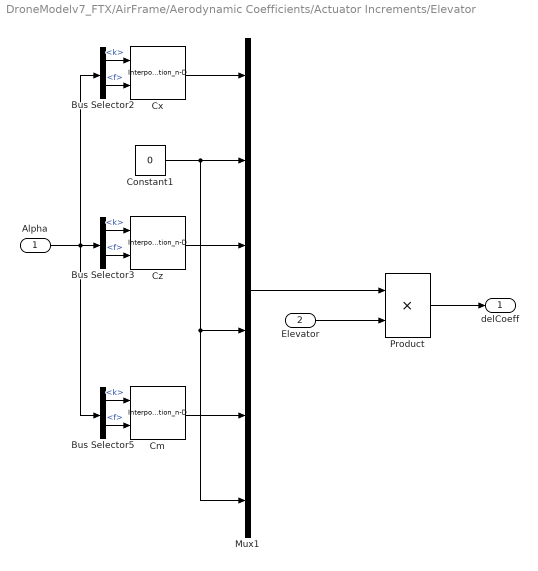
== system DroneModelv7_FTX/AirFrame/Aerodynamic Coefficients/Actuator Increments/Elevator ==
  Alpha : Inport
  Elevator : Inport  Port=2
  Bus Selector2 : BusSelector  OutputSignals=k,f
  Bus Selector3 : BusSelector  OutputSignals=k,f
  Bus Selector5 : BusSelector  OutputSignals=k,f
  Cm : Interpolation_n-D  NumberOfTableDimensions=1  Table=Cmde  RemoveProtectionIndex=on  SaturateOnIntegerOverflow=on
      settings: InputPortMap=u0,u1
  Constant1 : Constant  Value=0
  Cx : Interpolation_n-D  NumberOfTableDimensions=1  Table=CXde  RemoveProtectionIndex=on  SaturateOnIntegerOverflow=on
      settings: InputPortMap=u0,u1
  Cz : Interpolation_n-D  NumberOfTableDimensions=1  Table=CZde  RemoveProtectionIndex=on  SaturateOnIntegerOverflow=on
      settings: InputPortMap=u0,u1
  Mux1 : Mux  Inputs=6
  Product : Product  InputSameDT=on  SaturateOnIntegerOverflow=on  OutDataTypeStr=Inherit: Same as first input
  delCoeff : Outport  VectorParamsAs1DForOutWhenUnconnected=off
  wires:
  Bus Selector5/2 -> Cm/2  "<f>"
  Bus Selector5/1 -> Cm/1  "<k>"
  Bus Selector3/2 -> Cz/2  "<f>"
  Bus Selector3/1 -> Cz/1  "<k>"
  Bus Selector2/2 -> Cx/2  "<f>"
  Bus Selector2/1 -> Cx/1  "<k>"
  Constant1/1 -> Mux1/6, Mux1/4, Mux1/2
  Cm/1 -> Mux1/5
  Cz/1 -> Mux1/3
  Cx/1 -> Mux1/1
  Alpha/1 -> Bus Selector5/1, Bus Selector3/1, Bus Selector2/1
  Mux1/1 -> Product/1
  Product/1 -> delCoeff/1
  Elevator/1 -> Product/2

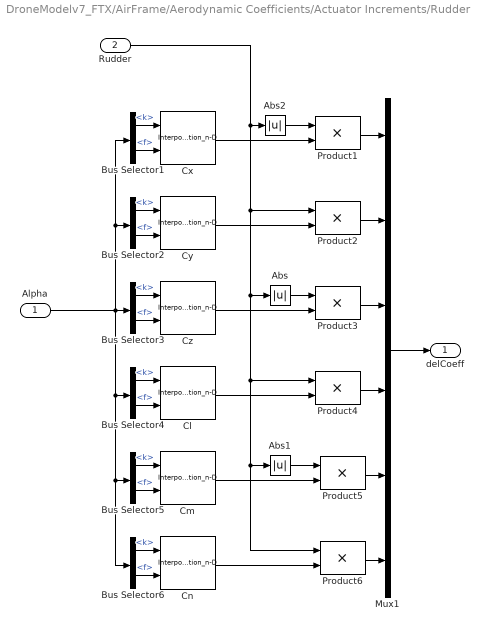
== system DroneModelv7_FTX/AirFrame/Aerodynamic Coefficients/Actuator Increments/Rudder ==
  Alpha : Inport
  Rudder : Inport  Port=2
  Abs : Abs
  Abs1 : Abs
  Abs2 : Abs
  Bus Selector{1..6} (6 alike) : BusSelector  OutputSignals=k,f
  Cl : Interpolation_n-D  NumberOfTableDimensions=1  Table=Cldr  RemoveProtectionIndex=on  SaturateOnIntegerOverflow=on
      settings: InputPortMap=u0,u1
  Cm : Interpolation_n-D  NumberOfTableDimensions=1  Table=Cmdr  RemoveProtectionIndex=on  SaturateOnIntegerOverflow=on
      settings: InputPortMap=u0,u1
  Cn : Interpolation_n-D  NumberOfTableDimensions=1  Table=Cndr  RemoveProtectionIndex=on  SaturateOnIntegerOverflow=on
      settings: InputPortMap=u0,u1
  Cx : Interpolation_n-D  NumberOfTableDimensions=1  Table=CXdr  RemoveProtectionIndex=on  SaturateOnIntegerOverflow=on
      settings: InputPortMap=u0,u1
  Cy : Interpolation_n-D  NumberOfTableDimensions=1  Table=CYdr  RemoveProtectionIndex=on  SaturateOnIntegerOverflow=on
      settings: InputPortMap=u0,u1
  Cz : Interpolation_n-D  NumberOfTableDimensions=1  Table=CZdr  RemoveProtectionIndex=on  SaturateOnIntegerOverflow=on
      settings: InputPortMap=u0,u1
  Mux1 : Mux  Inputs=6
  Product{1..6} (6 alike) : Product  InputSameDT=on  SaturateOnIntegerOverflow=on  OutDataTypeStr=Inherit: Same as first input
  delCoeff : Outport  VectorParamsAs1DForOutWhenUnconnected=off
  wires:
  Mux1/1 -> delCoeff/1
  Product1/1 -> Mux1/1
  Cx/1 -> Product1/2
  Product2/1 -> Mux1/2
  Cy/1 -> Product2/2
  Product3/1 -> Mux1/3
  Cz/1 -> Product3/2
  Cl/1 -> Product4/2
  Product4/1 -> Mux1/4
  Cm/1 -> Product5/2
  Product5/1 -> Mux1/5
  Cn/1 -> Product6/2
  Product6/1 -> Mux1/6
  Rudder/1 -> Product6/1, Abs1/1, Product4/1, Abs/1, Product2/1, Abs2/1
  Abs/1 -> Product3/1
  Abs1/1 -> Product5/1
  Abs2/1 -> Product1/1
  Alpha/1 -> Bus Selector1/1, Bus Selector2/1, Bus Selector5/1, Bus Selector6/1, Bus Selector4/1, Bus Selector3/1
  Bus Selector1/1 -> Cx/1  "<k>"
  Bus Selector1/2 -> Cx/2  "<f>"
  Bus Selector2/1 -> Cy/1  "<k>"
  Bus Selector2/2 -> Cy/2  "<f>"
  Bus Selector3/1 -> Cz/1  "<k>"
  Bus Selector3/2 -> Cz/2  "<f>"
  Bus Selector4/1 -> Cl/1  "<k>"
  Bus Selector4/2 -> Cl/2  "<f>"
  Bus Selector5/1 -> Cm/1  "<k>"
  Bus Selector5/2 -> Cm/2  "<f>"
  Bus Selector6/1 -> Cn/1  "<k>"
  Bus Selector6/2 -> Cn/2  "<f>"

== matlab function DroneModelv7_FTX/Sensors + Estimator/Sensor Models ==
  settings: updateMethod=DISCRETE  sampleTime=EST_TS
  data: pqr_t input; gyro_m output; acc_t input; Vb_t input; Ve_t input; SENS_P input; sb_in input; acc_m output; V_m output; Vz_m output; sb_out output
function [gyro_m, acc_m, V_m, Vz_m, sb_out] = fcn(pqr_t, acc_t, Vb_t, Ve_t, SENS_P, sb_in)
%#codegen
[gyro_m, acc_m, V_m, Vz_m, sb_out] = uav_sensors_step(pqr_t, acc_t, Vb_t, Ve_t, SENS_P, sb_in);
end

== matlab function DroneModelv7_FTX/Flight Control System/Controller/P phi ==
  data: alpha input; P output; beta input
function P = fcn(alpha,beta)

P = 0.05;

== matlab function DroneModelv7_FTX/Flight Control System/Controller/P alpha ==
  data: alpha input; P output; beta input
function P = fcn(alpha,beta)

P = 0.05;

== matlab function DroneModelv7_FTX/Flight Control System/Controller/P beta ==
  data: alpha input; P output; beta input
function P = fcn(alpha,beta)

P = -0.05;

== matlab function DroneModelv7_FTX/Sensors + Estimator/Estimator ==
  settings: updateMethod=DISCRETE  sampleTime=EST_TS
  data: gyro_m input; pqr_hat output; acc_m input; V_m input; Vz_m input; EST_P input; s_in input; alpha_hat output; beta_hat output; euler_hat output; s_out output
function [pqr_hat, alpha_hat, beta_hat, euler_hat, s_out] = fcn(gyro_m, acc_m, V_m, Vz_m, EST_P, s_in)
%#codegen
[pqr_hat, alpha_hat, beta_hat, euler_hat, s_out] = uav_estimator_step(gyro_m, acc_m, V_m, Vz_m, EST_P, s_in);
end

== matlab function DroneModelv7_FTX/Sensors + Estimator/Blend ==
  settings: updateMethod=DISCRETE  sampleTime=EST_TS
  data: pqr_h input; pqr_o output; alpha_h input; beta_h input; euler_h input; pqr_t input; alpha_t input; beta_t input; euler_t input; BL input; alpha_o output; beta_o output; euler_o output
function [pqr_o, alpha_o, beta_o, euler_o] = fcn(pqr_h, alpha_h, beta_h, euler_h, pqr_t, alpha_t, beta_t, euler_t, BL)
%#codegen
[pqr_o, alpha_o, beta_o, euler_o] = uav_blend_step(pqr_h, alpha_h, beta_h, euler_h, pqr_t, alpha_t, beta_t, euler_t, BL);
end

== matlab function DroneModelv7_FTX/AirFrame/Aerodynamic Coefficients/Damping Increments ==
  data: alpha_deg input; dC output; pqr input; V input; DMP_P input
function dC = damping(alpha_deg, pqr, V, DMP_P)
%#codegen
% Aerodynamic damping increments, [CX CY CZ Cl Cm Cn] in body axes.
% The HL-20 AirFrame terminates pqr and V and carries no damping at all.
dC = uav_damping_step(alpha_deg, pqr, V, DMP_P);
end
